simulink model "Questao_02"  (Simulink 7.1)
settings: Solver=ode45  StartTime=0.0  StopTime=300  RelTol=1e-3
InitFcn:
  | V=12;
  | R=50;
  | L=0.2;
  | 
  | KB=0.08;
  | KS=0.08;
  | KT=10;
  | K=100;
  | 
  | JM=8;
  | J2=4;
  | J3=20;
  | B1=0.2;
  | B2=0.4;
  | B3=0.8;
  | 
  | TREM_1_N1=10;
  | TREM_1_N2=50;
  | TREM_1_N3=10;
  | TREM_1_N4=20;
  | 
  | TREM_2_N1=10;
  | TREM_2_N2=80;
  | TREM_2_N3=40;
  | TREM_2_N4=50;
  | 
  | N1=TREM_1_N1;
  | N2=TREM_1_N2;
  | N3=TREM_1_N3;
  | N4=TREM_1_N4;
  | 
  | JEQ=JM+((N1/N2)^2)*J2+((N3/N4)^2)*((N1/N2)^2)*J3;
  | BEQ=B1+((N1/N2)^2)*B2+((N3/N4)^2)*((N1/N2)^2)*B3;
settings Model: Creator=ALUNO  LastModifiedBy=ALUNO
settings OptimizationCC: InlineInvariantSignals=on
settings DebuggingCC: SaveWithParameterizedLinksMsg=none  SignalResolutionControl=TryResolveAllWithWarning  MultiTaskDSMMsg=warning  MultiTaskCondExecSysMsg=none  StrictBusMsg=None
settings RTWCC: IncludeERTFirstTime=on
settings GRTTargetCC: TargetFcnLib=ansi_tfl_tmw.mat

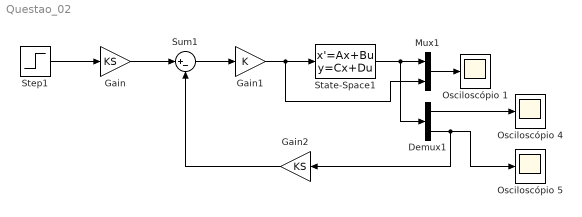
== system Questao_02 ==
  Demux1 : Demux  Outputs=2
  Gain : Gain  Gain=KS  ParameterDataType=sfix(16)  ParameterScaling=2^0  OutDataType=sfix(16)  OutScaling=2^0
  Gain1 : Gain  Gain=K  ParameterDataType=sfix(16)  ParameterScaling=2^0  OutDataType=sfix(16)  OutScaling=2^0
  Gain2 : Gain  Orientation=left  Gain=KS  ParameterDataType=sfix(16)  ParameterScaling=2^0  OutDataType=sfix(16)  OutScaling=2^0
  Mux1 : Mux  Inputs=2
  Osciloscópio 1 : Scope
      settings: TimeRange=70  YMin=0  YMax=10  MaxDataPoints=1000000
  Osciloscópio 4 : Scope
      settings: YMin=0  YMax=11  SaveName=ScopeData4  MaxDataPoints=1000000
  Osciloscópio 5 : Scope
      settings: YMin=0  YMax=11  SaveName=ScopeData5  MaxDataPoints=1000000
  State-Space1 : StateSpace  A=[-R/L,-KB/L,0;KT/JEQ,-BEQ/JEQ,0;0,1,0]  B=[1/L;0;0]  C=[0,(N1*N3)/(N2*N4),0;0,0,(N1*N3)/(N2*N4)]  D=[0;0]
  Step1 : Step  Time=0  After=V  SampleTime=0
  Sum1 : Sum  Inputs=|+-  OutDataType=sfix(16)  OutScaling=2^0
  wires:
  Mux1/1 -> Osciloscópio 1/1
  State-Space1/1 -> Mux1/1, Demux1/1
  Demux1/1 -> Osciloscópio 4/1
  Demux1/2 -> Osciloscópio 5/1, Gain2/1
  Step1/1 -> Gain/1
  Gain/1 -> Sum1/1
  Sum1/1 -> Gain1/1
  Gain1/1 -> State-Space1/1, Mux1/2
  Gain2/1 -> Sum1/2
